simulink model "sysball_plate"  (R2023a)
settings: Solver=VariableStepAuto  StartTime=0.0  StopTime=10.0  RelTol=1e-3
values from neighbouring files (symbols this model uses):
  A = [0 1 0 0 0 0; -c/J 0 0 0 k/J 0;0 0 0 1 0 0;0 0 -c/J 0 0 k/J;0 -k/l 0 0 -r/l 0;0 0 0 -k/l 0 -r/l]    [ball_plate_sys.m]    (also in ball_plate_sys2.m = [0 1 0 0 0;-c/J 0 k/J 0 0;0 -k/l -r/l 0 0;-1.96 0 0 0 0;0 0 )
  B = [b1 b2]    [ball_plate_sys.m]    (also in ball_plate_sys2.m = [0 0 -1 0 0]')
  C = [c1 ; c2]    [ball_plate_sys.m]    (also in ball_plate_sys2.m = [0 0 0 0 1])
  D = 0    [ball_plate_sys.m]    (also in ball_plate_sys2.m)
settings Model: Creator=Habib  LastModifiedBy=Habib

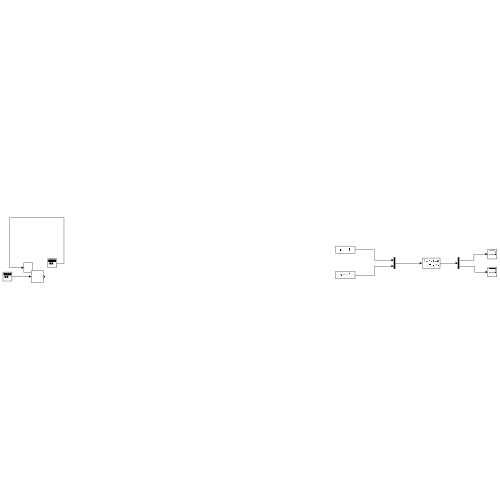
[thumbnail: Simulink's stored preview of the top-level diagram]
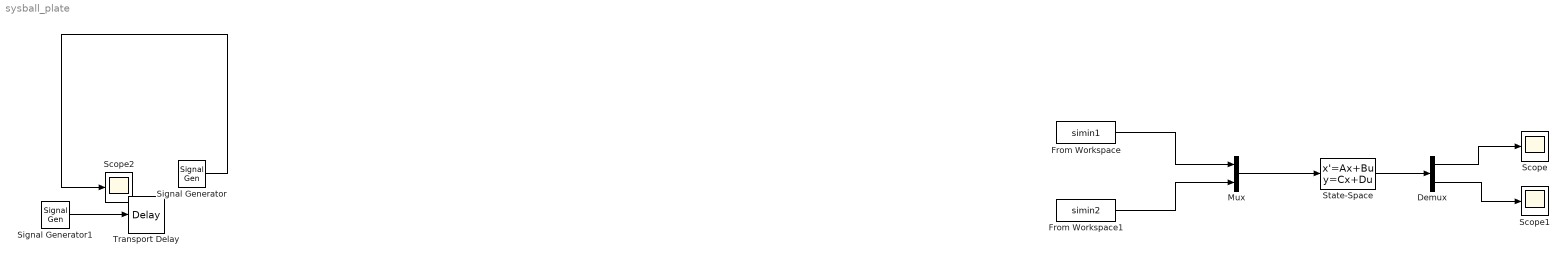
== system sysball_plate ==
  Demux : Demux  Outputs=2
  From Workspace : FromWorkspace  VariableName=simin1
  From Workspace1 : FromWorkspace  VariableName=simin2
  Mux : Mux  Inputs=2
  Scope : Scope
  Scope1 : Scope
  Scope2 : Scope
  Signal Generator : SignalGenerator  WaveForm=square  Units=rad/sec
  Signal Generator1 : SignalGenerator  WaveForm=square  Amplitude=2  Units=rad/sec
  State-Space : StateSpace  A=A  B=B  C=C  D=D  InitialCondition=0
  Transport Delay : TransportDelay
  wires:
  Signal Generator/1 -> Scope2/1
  Signal Generator1/1 -> Transport Delay/1
  State-Space/1 -> Demux/1
  Demux/1 -> Scope/1
  Demux/2 -> Scope1/1
  Mux/1 -> State-Space/1
  From Workspace/1 -> Mux/1
  From Workspace1/1 -> Mux/2
